simulink model "expert_control_model"  (R2022b)
settings: Solver=VariableStepAuto  StartTime=0.0  StopTime=1.6  RelTol=1e-3
libraries: slpidlib x4
settings Model: Creator=philf  LastModifiedBy=philf

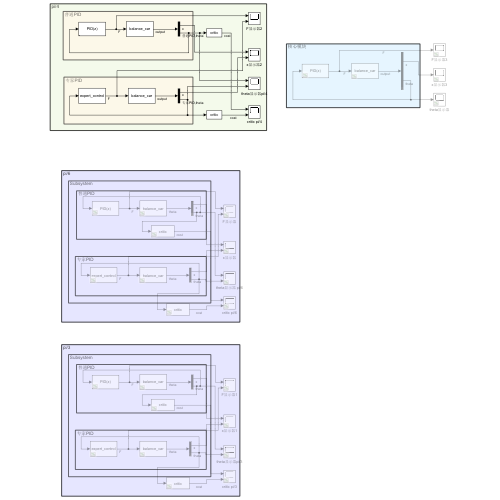
[thumbnail: Simulink's stored preview of the top-level diagram]
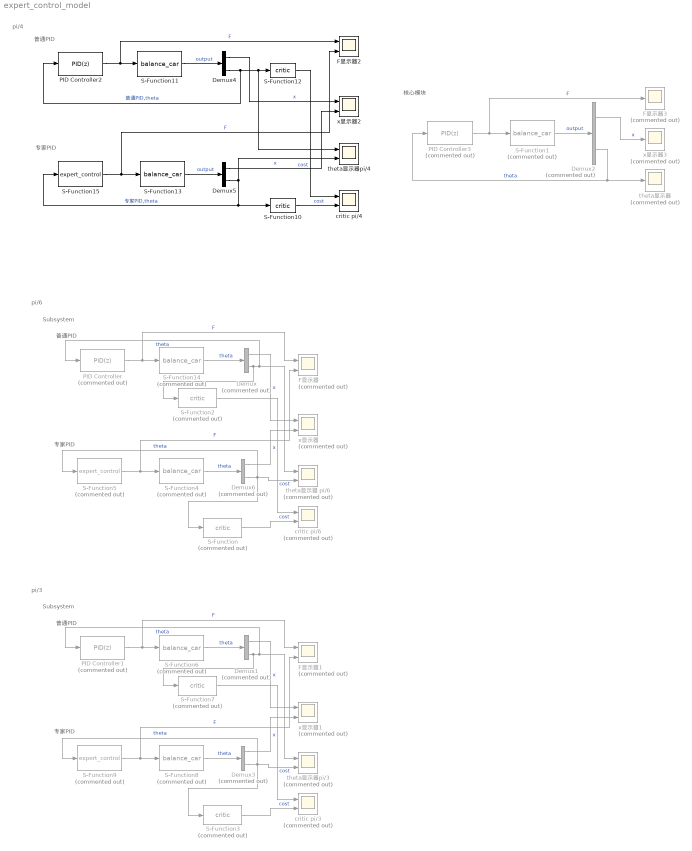
== system expert_control_model ==
  note: pi/6
  note: pi/4
  note: pi/3
  note: 专家PID
  note: 普通PID
  note: Subsystem
  note: 核心模块
  note: 普通PID
  note: 专家PID
  note: 专家PID
  note: 普通PID
  note: Subsystem
  Demux{,1..3,6} (5 alike) : Demux  Commented=on  Outputs=2
  Demux4 : Demux  Outputs=2
  Demux5 : Demux  Outputs=2
  F显示器 : Scope  Commented=on  NumInputPorts=2
  F显示器1 : Scope  Commented=on  NumInputPorts=2
  F显示器2 : Scope  NumInputPorts=2
  F显示器3 : Scope  Commented=on
  PID Controller : slpidlib/PID Controller  Commented=on  Controller=PID  Form=Parallel  TimeDomain=Discrete-time  UseExternalTs=off  SampleTime=0.0001  IntegratorMethod=Forward Euler  FilterMethod=Forward Euler  ControllerParametersSource=internal  P=200  I=0.001  UseKiTs=off  D=15  N=100  UseFilter=off  TunerSelectOption=Transfer Function Based (PID Tuner App)  InitialConditionSource=internal  InitialConditionForIntegrator=0  InitialConditionForFilter=0  DifferentiatorICPrevScaledInput=0  ExternalReset=none  TrackingMode=off  Kt=1  LimitOutput=off  SatLimitsSource=internal  UpperSaturationLimit=inf  LowerSaturationLimit=-inf  LinearizeAsGain=on  AntiWindupMode=none  Kb=1  LimitIntegrator=off  UpperIntegratorSaturationLimit=inf  LowerIntegratorSaturationLimit=-inf  POutMin=[]  POutMax=[]  IOutMin=[]  IOutMax=[]  DOutMin=[]  DOutMax=[]  NOutMin=[]  NOutMax=[]  SumOutMin=[]  SumOutMax=[]  SaturationOutMin=[]  SaturationOutMax=[]  PParamMin=[]  PParamMax=[]  IParamMin=[]  IParamMax=[]  DParamMin=[]  DParamMax=[]  NParamMin=[]  NParamMax=[]  KbParamMin=[]  KbParamMax=[]  KtParamMin=[]  KtParamMax=[]  KbOutMin=[]  KbOutMax=[]  KtOutMin=[]  KtOutMax=[]  IntegratorOutMin=[]  IntegratorOutMax=[]  FilterOutMin=[]  FilterOutMax=[]  SumI1OutMin=[]  SumI1OutMax=[]  SumI2OutMin=[]  SumI2OutMax=[]  SumI3OutMin=[]  SumI3OutMax=[]  SumI4OutMin=[]  SumI4OutMax=[]  SumDOutMin=[]  SumDOutMax=[]  DifferentiatorOutMin=[]  DifferentiatorOutMax=[]  FilterDiffOutCoefMin=[]  FilterDiffOutCoefMax=[]  ReciprocalOutMin=[]  ReciprocalOutMax=[]  SumDenOutMin=[]  SumDenOutMax=[]  SumNumOutMin=[]  SumNumOutMax=[]  DivideOutMin=[]  DivideOutMax=[]  UdiffTsProdOutMin=[]  UdiffTsProdOutMax=[]  NTsProdOutMin=[]  NTsProdOutMax=[]  UintegralTsProdOutMin=[]  UintegralTsProdOutMax=[]  UngainTsProdOutMin=[]  UngainTsProdOutMax=[]  ClampingZeroOutDataTypeStr=Inherit: Inherit via back propagation  ClampingZeroOutMin=[]  ClampingZeroOutMax=[]  FilterDenConstantOutDataTypeStr=Inherit: Inherit via back propagation  FilterDenConstantOutMin=[]  FilterDenConstantOutMax=[]  PCopyOutDataTypeStr=Inherit: Inherit via back propagation  PCopyOutMin=[]  PCopyOutMax=[]  NCopyOutDataTypeStr=Inherit: Inherit via back propagation  NCopyOutMin=[]  NCopyOutMax=[]  IntegratorContinuousStateAttributes=''  IntegratorStateMustResolveToSignalObject=off  IntegratorRTWStateStorageClass=Auto  FilterContinuousStateAttributes=''  FilterStateMustResolveToSignalObject=off  FilterRTWStateStorageClass=Auto  ParallelPVariant=InternalParameters  IdealPVariant=Disabled  IVariant=InternalParameters  DVariant=InternalParameters  IntegratorVariant=Discrete  SatVariant=Disabled  AWVariant=Passthrough  PCopyVariant=Disabled  TRVariant=Disabled  FdbkBlocksVariant=Forward  IdealPFdbkVariant=Disabled  SatFdbkVariant=Disabled  DerivativeFilterVariant=Differentiator  NVariant=Passthrough  NCopyVariant=Disabled_SignalSpec  FilterICVariant=InternalICsDifferentiator  IntegratorICVariant=InternalICs  ExternalResetVariant=Disabled  TRSumVariant=Passthrough  SumFdbkVariant=Disabled  SumVariant=Sum_PID  TsampFilterVariant=InternalTs  TsampNgainVariant=Passthrough  TsampIntegralVariant=Passthrough  ExternalSaturationOutDataTypeStr=Inherit: Same as second input
  PID Controller1 : slpidlib/PID Controller  Commented=on  Controller=PID  Form=Parallel  TimeDomain=Discrete-time  UseExternalTs=off  SampleTime=0.0001  IntegratorMethod=Forward Euler  FilterMethod=Forward Euler  ControllerParametersSource=internal  P=300  I=0.001  UseKiTs=off  D=15  N=100  UseFilter=off  TunerSelectOption=Transfer Function Based (PID Tuner App)  InitialConditionSource=internal  InitialConditionForIntegrator=0  InitialConditionForFilter=0  DifferentiatorICPrevScaledInput=0  ExternalReset=none  TrackingMode=off  Kt=1  LimitOutput=off  SatLimitsSource=internal  UpperSaturationLimit=inf  LowerSaturationLimit=-inf  LinearizeAsGain=on  AntiWindupMode=none  Kb=1  LimitIntegrator=off  UpperIntegratorSaturationLimit=inf  LowerIntegratorSaturationLimit=-inf  POutMin=[]  POutMax=[]  IOutMin=[]  IOutMax=[]  DOutMin=[]  DOutMax=[]  NOutMin=[]  NOutMax=[]  SumOutMin=[]  SumOutMax=[]  SaturationOutMin=[]  SaturationOutMax=[]  PParamMin=[]  PParamMax=[]  IParamMin=[]  IParamMax=[]  DParamMin=[]  DParamMax=[]  NParamMin=[]  NParamMax=[]  KbParamMin=[]  KbParamMax=[]  KtParamMin=[]  KtParamMax=[]  KbOutMin=[]  KbOutMax=[]  KtOutMin=[]  KtOutMax=[]  IntegratorOutMin=[]  IntegratorOutMax=[]  FilterOutMin=[]  FilterOutMax=[]  SumI1OutMin=[]  SumI1OutMax=[]  SumI2OutMin=[]  SumI2OutMax=[]  SumI3OutMin=[]  SumI3OutMax=[]  SumI4OutMin=[]  SumI4OutMax=[]  SumDOutMin=[]  SumDOutMax=[]  DifferentiatorOutMin=[]  DifferentiatorOutMax=[]  FilterDiffOutCoefMin=[]  FilterDiffOutCoefMax=[]  ReciprocalOutMin=[]  ReciprocalOutMax=[]  SumDenOutMin=[]  SumDenOutMax=[]  SumNumOutMin=[]  SumNumOutMax=[]  DivideOutMin=[]  DivideOutMax=[]  UdiffTsProdOutMin=[]  UdiffTsProdOutMax=[]  NTsProdOutMin=[]  NTsProdOutMax=[]  UintegralTsProdOutMin=[]  UintegralTsProdOutMax=[]  UngainTsProdOutMin=[]  UngainTsProdOutMax=[]  ClampingZeroOutDataTypeStr=Inherit: Inherit via back propagation  ClampingZeroOutMin=[]  ClampingZeroOutMax=[]  FilterDenConstantOutDataTypeStr=Inherit: Inherit via back propagation  FilterDenConstantOutMin=[]  FilterDenConstantOutMax=[]  PCopyOutDataTypeStr=Inherit: Inherit via back propagation  PCopyOutMin=[]  PCopyOutMax=[]  NCopyOutDataTypeStr=Inherit: Inherit via back propagation  NCopyOutMin=[]  NCopyOutMax=[]  IntegratorContinuousStateAttributes=''  IntegratorStateMustResolveToSignalObject=off  IntegratorRTWStateStorageClass=Auto  FilterContinuousStateAttributes=''  FilterStateMustResolveToSignalObject=off  FilterRTWStateStorageClass=Auto  ParallelPVariant=InternalParameters  IdealPVariant=Disabled  IVariant=InternalParameters  DVariant=InternalParameters  IntegratorVariant=Discrete  SatVariant=Disabled  AWVariant=Passthrough  PCopyVariant=Disabled  TRVariant=Disabled  FdbkBlocksVariant=Forward  IdealPFdbkVariant=Disabled  SatFdbkVariant=Disabled  DerivativeFilterVariant=Differentiator  NVariant=Passthrough  NCopyVariant=Disabled_SignalSpec  FilterICVariant=InternalICsDifferentiator  IntegratorICVariant=InternalICs  ExternalResetVariant=Disabled  TRSumVariant=Passthrough  SumFdbkVariant=Disabled  SumVariant=Sum_PID  TsampFilterVariant=InternalTs  TsampNgainVariant=Passthrough  TsampIntegralVariant=Passthrough  ExternalSaturationOutDataTypeStr=Inherit: Same as second input
  PID Controller2 : slpidlib/PID Controller  Controller=PID  Form=Parallel  TimeDomain=Discrete-time  UseExternalTs=off  SampleTime=0.0001  IntegratorMethod=Forward Euler  FilterMethod=Forward Euler  ControllerParametersSource=internal  P=200  I=0.001  UseKiTs=off  D=10  N=100  UseFilter=off  TunerSelectOption=Transfer Function Based (PID Tuner App)  InitialConditionSource=internal  InitialConditionForIntegrator=0  InitialConditionForFilter=0  DifferentiatorICPrevScaledInput=0  ExternalReset=none  TrackingMode=off  Kt=1  LimitOutput=off  SatLimitsSource=internal  UpperSaturationLimit=inf  LowerSaturationLimit=-inf  LinearizeAsGain=on  AntiWindupMode=none  Kb=1  LimitIntegrator=off  UpperIntegratorSaturationLimit=inf  LowerIntegratorSaturationLimit=-inf  POutMin=[]  POutMax=[]  IOutMin=[]  IOutMax=[]  DOutMin=[]  DOutMax=[]  NOutMin=[]  NOutMax=[]  SumOutMin=[]  SumOutMax=[]  SaturationOutMin=[]  SaturationOutMax=[]  PParamMin=[]  PParamMax=[]  IParamMin=[]  IParamMax=[]  DParamMin=[]  DParamMax=[]  NParamMin=[]  NParamMax=[]  KbParamMin=[]  KbParamMax=[]  KtParamMin=[]  KtParamMax=[]  KbOutMin=[]  KbOutMax=[]  KtOutMin=[]  KtOutMax=[]  IntegratorOutMin=[]  IntegratorOutMax=[]  FilterOutMin=[]  FilterOutMax=[]  SumI1OutMin=[]  SumI1OutMax=[]  SumI2OutMin=[]  SumI2OutMax=[]  SumI3OutMin=[]  SumI3OutMax=[]  SumI4OutMin=[]  SumI4OutMax=[]  SumDOutMin=[]  SumDOutMax=[]  DifferentiatorOutMin=[]  DifferentiatorOutMax=[]  FilterDiffOutCoefMin=[]  FilterDiffOutCoefMax=[]  ReciprocalOutMin=[]  ReciprocalOutMax=[]  SumDenOutMin=[]  SumDenOutMax=[]  SumNumOutMin=[]  SumNumOutMax=[]  DivideOutMin=[]  DivideOutMax=[]  UdiffTsProdOutMin=[]  UdiffTsProdOutMax=[]  NTsProdOutMin=[]  NTsProdOutMax=[]  UintegralTsProdOutMin=[]  UintegralTsProdOutMax=[]  UngainTsProdOutMin=[]  UngainTsProdOutMax=[]  ClampingZeroOutDataTypeStr=Inherit: Inherit via back propagation  ClampingZeroOutMin=[]  ClampingZeroOutMax=[]  FilterDenConstantOutDataTypeStr=Inherit: Inherit via back propagation  FilterDenConstantOutMin=[]  FilterDenConstantOutMax=[]  PCopyOutDataTypeStr=Inherit: Inherit via back propagation  PCopyOutMin=[]  PCopyOutMax=[]  NCopyOutDataTypeStr=Inherit: Inherit via back propagation  NCopyOutMin=[]  NCopyOutMax=[]  IntegratorContinuousStateAttributes=''  IntegratorStateMustResolveToSignalObject=off  IntegratorRTWStateStorageClass=Auto  FilterContinuousStateAttributes=''  FilterStateMustResolveToSignalObject=off  FilterRTWStateStorageClass=Auto  ParallelPVariant=InternalParameters  IdealPVariant=Disabled  IVariant=InternalParameters  DVariant=InternalParameters  IntegratorVariant=Discrete  SatVariant=Disabled  AWVariant=Passthrough  PCopyVariant=Disabled  TRVariant=Disabled  FdbkBlocksVariant=Forward  IdealPFdbkVariant=Disabled  SatFdbkVariant=Disabled  DerivativeFilterVariant=Differentiator  NVariant=Passthrough  NCopyVariant=Disabled_SignalSpec  FilterICVariant=InternalICsDifferentiator  IntegratorICVariant=InternalICs  ExternalResetVariant=Disabled  TRSumVariant=Passthrough  SumFdbkVariant=Disabled  SumVariant=Sum_PID  TsampFilterVariant=InternalTs  TsampNgainVariant=Passthrough  TsampIntegralVariant=Passthrough  ExternalSaturationOutDataTypeStr=Inherit: Same as second input
  PID Controller3 : slpidlib/PID Controller  Commented=on  Controller=PID  Form=Parallel  TimeDomain=Discrete-time  UseExternalTs=off  SampleTime=0.0001  IntegratorMethod=Forward Euler  FilterMethod=Forward Euler  ControllerParametersSource=internal  P=200  I=0.001  UseKiTs=off  D=10  N=100  UseFilter=off  TunerSelectOption=Transfer Function Based (PID Tuner App)  InitialConditionSource=internal  InitialConditionForIntegrator=0  InitialConditionForFilter=0  DifferentiatorICPrevScaledInput=0  ExternalReset=none  TrackingMode=off  Kt=1  LimitOutput=off  SatLimitsSource=internal  UpperSaturationLimit=inf  LowerSaturationLimit=-inf  LinearizeAsGain=on  AntiWindupMode=none  Kb=1  LimitIntegrator=off  UpperIntegratorSaturationLimit=inf  LowerIntegratorSaturationLimit=-inf  POutMin=[]  POutMax=[]  IOutMin=[]  IOutMax=[]  DOutMin=[]  DOutMax=[]  NOutMin=[]  NOutMax=[]  SumOutMin=[]  SumOutMax=[]  SaturationOutMin=[]  SaturationOutMax=[]  PParamMin=[]  PParamMax=[]  IParamMin=[]  IParamMax=[]  DParamMin=[]  DParamMax=[]  NParamMin=[]  NParamMax=[]  KbParamMin=[]  KbParamMax=[]  KtParamMin=[]  KtParamMax=[]  KbOutMin=[]  KbOutMax=[]  KtOutMin=[]  KtOutMax=[]  IntegratorOutMin=[]  IntegratorOutMax=[]  FilterOutMin=[]  FilterOutMax=[]  SumI1OutMin=[]  SumI1OutMax=[]  SumI2OutMin=[]  SumI2OutMax=[]  SumI3OutMin=[]  SumI3OutMax=[]  SumI4OutMin=[]  SumI4OutMax=[]  SumDOutMin=[]  SumDOutMax=[]  DifferentiatorOutMin=[]  DifferentiatorOutMax=[]  FilterDiffOutCoefMin=[]  FilterDiffOutCoefMax=[]  ReciprocalOutMin=[]  ReciprocalOutMax=[]  SumDenOutMin=[]  SumDenOutMax=[]  SumNumOutMin=[]  SumNumOutMax=[]  DivideOutMin=[]  DivideOutMax=[]  UdiffTsProdOutMin=[]  UdiffTsProdOutMax=[]  NTsProdOutMin=[]  NTsProdOutMax=[]  UintegralTsProdOutMin=[]  UintegralTsProdOutMax=[]  UngainTsProdOutMin=[]  UngainTsProdOutMax=[]  ClampingZeroOutDataTypeStr=Inherit: Inherit via back propagation  ClampingZeroOutMin=[]  ClampingZeroOutMax=[]  FilterDenConstantOutDataTypeStr=Inherit: Inherit via back propagation  FilterDenConstantOutMin=[]  FilterDenConstantOutMax=[]  PCopyOutDataTypeStr=Inherit: Inherit via back propagation  PCopyOutMin=[]  PCopyOutMax=[]  NCopyOutDataTypeStr=Inherit: Inherit via back propagation  NCopyOutMin=[]  NCopyOutMax=[]  IntegratorContinuousStateAttributes=''  IntegratorStateMustResolveToSignalObject=off  IntegratorRTWStateStorageClass=Auto  FilterContinuousStateAttributes=''  FilterStateMustResolveToSignalObject=off  FilterRTWStateStorageClass=Auto  ParallelPVariant=InternalParameters  IdealPVariant=Disabled  IVariant=InternalParameters  DVariant=InternalParameters  IntegratorVariant=Discrete  SatVariant=Disabled  AWVariant=Passthrough  PCopyVariant=Disabled  TRVariant=Disabled  FdbkBlocksVariant=Forward  IdealPFdbkVariant=Disabled  SatFdbkVariant=Disabled  DerivativeFilterVariant=Differentiator  NVariant=Passthrough  NCopyVariant=Disabled_SignalSpec  FilterICVariant=InternalICsDifferentiator  IntegratorICVariant=InternalICs  ExternalResetVariant=Disabled  TRSumVariant=Passthrough  SumFdbkVariant=Disabled  SumVariant=Sum_PID  TsampFilterVariant=InternalTs  TsampNgainVariant=Passthrough  TsampIntegralVariant=Passthrough  ExternalSaturationOutDataTypeStr=Inherit: Same as second input
  S-Function{,2..3,7} (4 alike) : S-Function  Commented=on  FunctionName=critic  SFunctionDeploymentMode=off  EnableBusSupport=off
  S-Function1 : S-Function  Commented=on  FunctionName=balance_car  Parameters=angle  SFunctionDeploymentMode=off  EnableBusSupport=off  mask{angle=pi/4}
      mask prompts: angle "初始角度"
      mask DialogControl ParameterGroupVar Prompt: 参数
  S-Function10 : S-Function  FunctionName=critic  SFunctionDeploymentMode=off  EnableBusSupport=off
  S-Function11 : S-Function  FunctionName=balance_car  Parameters=angle  SFunctionDeploymentMode=off  EnableBusSupport=off  mask{angle=pi/4}
      mask prompts: angle "初始角度"
      mask DialogControl ParameterGroupVar Prompt: 参数
  S-Function12 : S-Function  FunctionName=critic  SFunctionDeploymentMode=off  EnableBusSupport=off
  S-Function13 : S-Function  FunctionName=balance_car  Parameters=angle  SFunctionDeploymentMode=off  EnableBusSupport=off  mask{angle=pi/4}
      mask prompts: angle "初始角度"
      mask DialogControl ParameterGroupVar Prompt: 参数
  S-Function14 : S-Function  Commented=on  FunctionName=balance_car  Parameters=angle  SFunctionDeploymentMode=off  EnableBusSupport=off  mask{angle=pi/6}
      mask prompts: angle "初始角度"
      mask DialogControl ParameterGroupVar Prompt: 参数
  S-Function15 : S-Function  FunctionName=expert_control  Parameters=K_b,K_s,theta_m,theta_2,theta_1,Kp,Ki,Kd,pi/4,F_m  SFunctionDeploymentMode=off  EnableBusSupport=off  mask{K_b=2.4, K_s=0.5, theta_m=0.6, theta_2=0.2, theta_1=0.05, Kp=200, Ki=0.001, Kd=20, angle=pi/4, F_m=28}
      mask prompts: Kp "PID-Kp"; Ki "PID-Ki"; Kd "PID-Kd"; angle "初始角度"; F_m "最大外力"
      mask DialogControl ParameterGroupVar Prompt: 参数
  S-Function4 : S-Function  Commented=on  FunctionName=balance_car  Parameters=angle  SFunctionDeploymentMode=off  EnableBusSupport=off  mask{angle=pi/6}
      mask prompts: angle "初始角度"
      mask DialogControl ParameterGroupVar Prompt: 参数
  S-Function5 : S-Function  Commented=on  FunctionName=expert_control  Parameters=K_b,K_s,theta_m,theta_2,theta_1,Kp,Ki,Kd,pi/4,F_m  SFunctionDeploymentMode=off  EnableBusSupport=off  mask{K_b=7, K_s=0.9, theta_m=0.5, theta_2=0.25, theta_1=0.1, Kp=200, Ki=0.001, Kd=20, angle=pi/6, F_m=30}
      mask prompts: Kp "PID-Kp"; Ki "PID-Ki"; Kd "PID-Kd"; angle "初始角度"; F_m "最大外力"
      mask DialogControl ParameterGroupVar Prompt: 参数
  S-Function6 : S-Function  Commented=on  FunctionName=balance_car  Parameters=angle  SFunctionDeploymentMode=off  EnableBusSupport=off  mask{angle=pi/3}
      mask prompts: angle "初始角度"
      mask DialogControl ParameterGroupVar Prompt: 参数
  S-Function8 : S-Function  Commented=on  FunctionName=balance_car  Parameters=angle  SFunctionDeploymentMode=off  EnableBusSupport=off  mask{angle=pi/3}
      mask prompts: angle "初始角度"
      mask DialogControl ParameterGroupVar Prompt: 参数
  S-Function9 : S-Function  Commented=on  FunctionName=expert_control  Parameters=K_b,K_s,theta_m,theta_2,theta_1,Kp,Ki,Kd,pi/4,F_m  SFunctionDeploymentMode=off  EnableBusSupport=off  mask{K_b=8, K_s=0.95, theta_m=0.8, theta_2=0.5, theta_1=0.20, Kp=300, Ki=0.001, Kd=15, angle=pi/3, F_m=100}
      mask prompts: Kp "PID-Kp"; Ki "PID-Ki"; Kd "PID-Kd"; angle "初始角度"; F_m "最大外力"
      mask DialogControl ParameterGroupVar Prompt: 参数
  critic pi/3 : Scope  Commented=on  NumInputPorts=2
  critic pi/4 : Scope  NumInputPorts=2
  critic pi/6 : Scope  Commented=on  NumInputPorts=2
  theta显示器 : Scope  Commented=on
  theta显示器 pi/6 : Scope  Commented=on  NumInputPorts=2
  theta显示器pi/3 : Scope  Commented=on  NumInputPorts=2
  theta显示器pi/4 : Scope  NumInputPorts=2
  x显示器 : Scope  Commented=on  NumInputPorts=2
  x显示器1 : Scope  Commented=on  NumInputPorts=2
  x显示器2 : Scope  NumInputPorts=2
  x显示器3 : Scope  Commented=on
  wires:
  Demux1/1 -> x显示器1/1  "x"
  S-Function3/1 -> critic pi/3/2  "cost"
  PID Controller1/1 -> F显示器1/1, S-Function6/1  "F"
  S-Function9/1 -> F显示器1/2, S-Function8/1  "F"
  S-Function7/1 -> critic pi/3/1  "cost"
  Demux3/1 -> x显示器1/2  "x"
  S-Function8/1 -> Demux3/1  "theta"
  S-Function6/1 -> Demux1/1  "theta"
  Demux3/2 -> S-Function9/1, S-Function3/1, theta显示器pi/3/2  "theta"
  Demux1/2 -> S-Function7/1, theta显示器pi/3/1, PID Controller1/1  "theta"
  Demux2/1 -> x显示器3/1  "x"
  PID Controller3/1 -> S-Function1/1, F显示器3/1  "F"
  S-Function1/1 -> Demux2/1  "output"
  Demux2/2 -> PID Controller3/1, theta显示器/1  "theta"
  S-Function12/1 -> critic pi/4/1  "cost"
  S-Function10/1 -> critic pi/4/2  "cost"
  Demux4/1 -> x显示器2/1  "x"
  S-Function13/1 -> Demux5/1  "output"
  Demux5/2 -> S-Function15/1, S-Function10/1, theta显示器pi/4/2  "专家PID,theta"
  PID Controller2/1 -> F显示器2/1, S-Function11/1  "F"
  S-Function11/1 -> Demux4/1  "output"
  S-Function15/1 -> F显示器2/2, S-Function13/1  "F"
  Demux5/1 -> x显示器2/2  "x"
  Demux4/2 -> theta显示器pi/4/1, S-Function12/1, PID Controller2/1  "普通PID,theta"
  S-Function14/1 -> Demux/1  "theta"
  S-Function5/1 -> F显示器/2, S-Function4/1  "F"
  Demux/2 -> S-Function2/1, theta显示器 pi/6/1, PID Controller/1  "theta"
  S-Function2/1 -> critic pi/6/1  "cost"
  Demux/1 -> x显示器/1  "x"
  PID Controller/1 -> F显示器/1, S-Function14/1  "F"
  S-Function/1 -> critic pi/6/2  "cost"
  Demux6/1 -> x显示器/2  "x"
  Demux6/2 -> S-Function/1, theta显示器 pi/6/2, S-Function5/1  "theta"
  S-Function4/1 -> Demux6/1  "theta"
